simulink model "induction_motor_speedcontrol"  (R2021a)
settings: Solver=ode23t  StartTime=0.0  StopTime=2  RelTol=1e-3
libraries: spsRMSLib x3, spsVoltageMeasurementLib x3, spsDCVoltageSourceLib x1, spsAsynchronousMachineSIUnitsLib x1, spsPWMGenerator2LevelLib x1, spsUniversalBridgeLib x1, spspowerguiLib x1
settings Model: Creator=Davie  LastModifiedBy=Davie

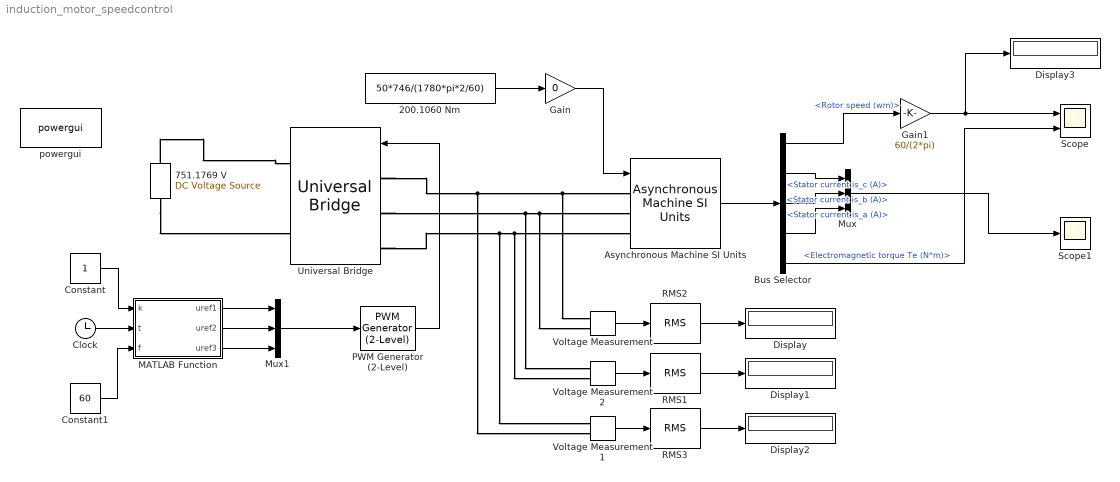
== system induction_motor_speedcontrol ==
  200.1060 Nm : Constant  Value=50*746/(1780*pi*2/60)
  751.1769 V : spsDCVoltageSourceLib/DC Voltage Source  Amplitude=460/sqrt(3)*sqrt(2)*2  Measurements=None
  Asynchronous Machine SI Units : spsAsynchronousMachineSIUnitsLib/Asynchronous Machine SI Units  RotorType=Squirrel-cage  PresetModel="04:  50 HP  460 V 60Hz 1780 RPM"  MechanicalLoad=Torque Tm  ShowDetailedParameters=on  ReferenceFrame=Rotor  Units=SI  MeasurementBus=off  NominalParameters=[3.73e+04 460 60]  VoltageRatio=1  Stator=[0.09961 0.000867]  Rotor=[0.05837 0.000867]  Cage1=[0.4155 0.002066]  Cage2=[0.4168 0.0003495]  Lm=0.03039  Mechanical=[0.4 0.02187 2]  PolePairs=2  InitialConditions=[1 0 0 0 0 0 0 0]  SimulateSaturation=off  Saturation=[14.03593122, 27.81365428, 53.79336849, 72.68890987, 97.98006896, 148.6815601, 215.7428561, 302.9841135, 428.7778367 ; 230, 322, 414, 460, 506, 552, 598, 644, 690]  LoadFlowParameters=1492000  TsPowergui=0  TsBlock=-1  IterativeModel=Trapezoidal non iterative  IterativeDiscreteModel=Trapezoidal non iterative  Pmec=1.492e+006
  Bus Selector : BusSelector  OutputSignals=Mechanical.Rotor speed (wm),Stator measurements.Stator current is_c (A),Stator measurements.Stator current is_b (A),Stator measurements.Stator current is_a (A),Mechanical.Electromagnetic torque Te (N*m)
  Clock : Clock
  Constant : Constant
  Constant1 : Constant  Value=60
  Display{,1..3} (4 alike) : Display
  Gain : Gain  Gain=0
  Gain1 : Gain  Gain=60/(2*pi)
  MATLAB Function : MATLAB Function  TreatAsAtomicUnit=on
  Mux : Mux  Inputs=3
  Mux1 : Mux  Inputs=3
  PWM Generator (2-Level) : spsPWMGenerator2LevelLib/PWM Generator (2-Level)  ModulatorType=Three-phase bridge (6 pulses)  ModulatorMode=Unsynchronized  Fc=200*60  Pc=90  nF=27  MinMax="[ -1  1 ]"  SamplingTechnique=Natural  ModulatingSignals=off  m=0.8  Freq=60  Phase=0  Ts=0  ShowCarrierOutport=off
  RMS1 : spsRMSLib/RMS  TrueRMS=off  Freq=60  RMSInit=120  Ts=0
  RMS2 : spsRMSLib/RMS  TrueRMS=off  Freq=60  RMSInit=120  Ts=0
  RMS3 : spsRMSLib/RMS  TrueRMS=on  Freq=60  RMSInit=120  Ts=0
  Scope : Scope  NumInputPorts=2
  Scope1 : Scope
  Universal Bridge : spsUniversalBridgeLib/Universal Bridge  Arms=3  SnubberResistance=1e5  SnubberCapacitance=inf  Device=IGBT / Diodes  Ron=1e-3  Lon=0  ForwardVoltages="[  0  0  ]"  ForwardVoltage=0  GTOparameters=[ 10e-6 , 20e-6 ]  IGBTparameters=[ 1e-6 , 2e-6 ]  Measurements=None  Measurements_2=None  converterType=Rectifier
  Voltage Measurement : spsVoltageMeasurementLib/Voltage Measurement  PhasorSimulation=off  OutputType=Complex  PSBequivalent=0
  Voltage Measurement1 : spsVoltageMeasurementLib/Voltage Measurement  PhasorSimulation=off  OutputType=Complex  PSBequivalent=0
  Voltage Measurement2 : spsVoltageMeasurementLib/Voltage Measurement  PhasorSimulation=off  OutputType=Complex  PSBequivalent=0
  powergui : spspowerguiLib/powergui  Priority=1  SimulationMode=Continuous  SampleTime=50e-6  frequency=60  Iterations=50  frequencyindice=60  Pbase=100e6  ErrMax=1e-4  UnitsV=kV  UnitsW=MW  buscounter=0  FunctionMessages=off  echomessages=off  EnableUseOfTLC=off  CurrentSourceSwitches=off  DisableSnubberDevices=off  DisableRonSwitches=off  DisableVfSwitches=off  DisplayEquations=off  AutomaticDiscreteSolvers=off  SolverType=Tustin/Backward Euler (TBE)  Interpol=off  ExternalGateDelay=off  methode=off  Ts=100  x0status=blocks  SPID=on  SwTol=0  HookPort=off  NonlinearTolerance=1e-4  nMaxIteration=100  ContinueOnMaxIteration=off  RestoreLinks=warning  ResistiveCurrentMeasurement=off  Frange=[0:2:500]  Ylog=off  Xlog=on  ShowGrid=off  save=off  variable=ZData  structure=0  ZoomFFT=off  StartTime=0.0  cycles=1  DisplayStyle=1  fundamental=60  FreqAxis=off  MaxFrequency=1000  frequencyindicesteady=1  RmsSteady=1  display=off
  wires:
  200.1060 Nm/1 -> Gain/1
  Gain/1 -> Asynchronous Machine SI Units/1
  Asynchronous Machine SI Units/1 -> Bus Selector/1
  Bus Selector/1 -> Gain1/1  "<Rotor speed (wm)>"
  Bus Selector/5 -> Scope/2  "<Electromagnetic torque Te (N*m)>"
  Bus Selector/2 -> Mux/1  "<Stator current is_c (A)>"
  Bus Selector/3 -> Mux/2  "<Stator current is_b (A)>"
  Bus Selector/4 -> Mux/3  "<Stator current is_a (A)>"
  Mux/1 -> Scope1/1
  Gain1/1 -> Display3/1, Scope/1
  PWM Generator (2-Level)/1 -> Universal Bridge/1
  MATLAB Function/2(uref2) -> Mux1/2
  MATLAB Function/3(uref3) -> Mux1/3
  MATLAB Function/1(uref1) -> Mux1/1
  Mux1/1 -> PWM Generator (2-Level)/1
  Constant/1 -> MATLAB Function/1(k)
  Clock/1 -> MATLAB Function/2(t)
  Constant1/1 -> MATLAB Function/3(f)
  Voltage Measurement/1 -> RMS2/1
  RMS2/1 -> Display/1
  Voltage Measurement2/1 -> RMS1/1
  RMS1/1 -> Display1/1
  Voltage Measurement1/1 -> RMS3/1
  RMS3/1 -> Display2/1
  connections:
  751.1769 V/RConn1 -- Universal Bridge/RConn1
  751.1769 V/LConn1 -- Universal Bridge/RConn2
  Universal Bridge/LConn1 -- Voltage Measurement1/LConn2 -- Voltage Measurement/LConn1 -- Asynchronous Machine SI Units/LConn1
  Universal Bridge/LConn2 -- Voltage Measurement2/LConn1 -- Voltage Measurement/LConn2 -- Asynchronous Machine SI Units/LConn2
  Universal Bridge/LConn3 -- Voltage Measurement1/LConn1 -- Voltage Measurement2/LConn2 -- Asynchronous Machine SI Units/LConn3

== matlab function induction_motor_speedcontrol/MATLAB Function ==
  data: k input; uref1 output; uref2 output; uref3 output; t input; f input
function [uref1, uref2, uref3]= fcn(k, t, f)
if t>0.5
    k=0.8
end
if t>1.2
    k=1
end    
uref1 = k*sin(2*pi*f*t*k);
uref2 = k*sin(2*pi*f*t*k - 2*pi/3);
uref3 = k*sin(2*pi*f*t*k + 2*pi/3);
end
